simulink model "Muscel_Model"  (R2016b)
settings: Solver=ode45  StartTime=0.0  StopTime=30  FixedStep=0.001  MinStep=0.0001  RelTol=1e-3
libraries: simulink x3
settings Model: Creator=Jan  LastModifiedBy=Jan

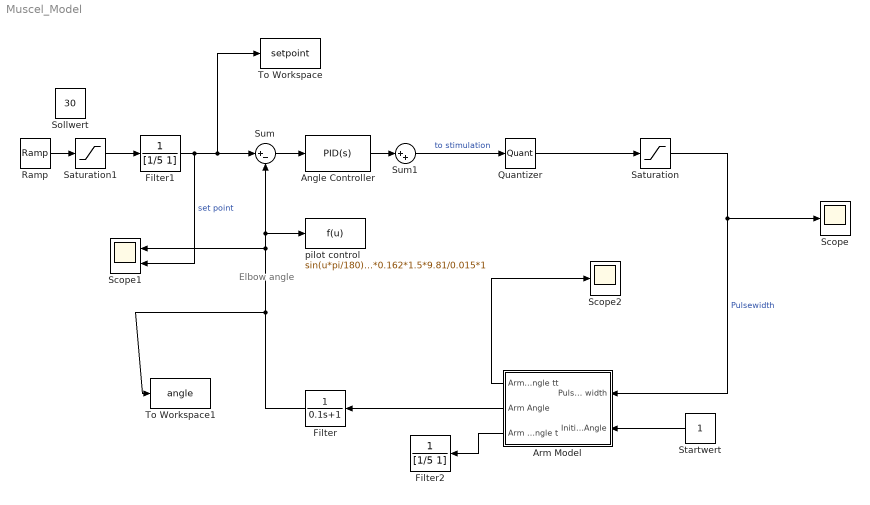
== system Muscel_Model ==
  note: Elbow angle
  Angle Controller : simulink/Continuous/PID Controller  Controller=PID  TimeDomain=Continuous-time  SampleTime=-1  IntegratorMethod=Forward Euler  FilterMethod=Forward Euler  Form=Parallel  UseFilter=on  ControllerParametersSource=internal  P=2  I=2  D=0.1  N=100  InitialConditionSource=internal  InitialConditionForIntegrator=0  InitialConditionForFilter=0  ExternalReset=none  LimitOutput=off  UpperSaturationLimit=500  LowerSaturationLimit=-inf  LinearizeAsGain=on  AntiWindupMode=none  Kb=1  TrackingMode=off  Kt=1  PParamMin=[]  PParamMax=[]  IParamMin=[]  IParamMax=[]  DParamMin=[]  DParamMax=[]  NParamMin=[]  NParamMax=[]  KbParamMin=[]  KbParamMax=[]  KtParamMin=[]  KtParamMax=[]  POutMin=[]  POutMax=[]  IOutMin=[]  IOutMax=[]  DOutMin=[]  DOutMax=[]  NOutMin=[]  NOutMax=[]  KbOutMin=[]  KbOutMax=[]  KtOutMin=[]  KtOutMax=[]  IntegratorOutMin=[]  IntegratorOutMax=[]  FilterOutMin=[]  FilterOutMax=[]  SumOutMin=[]  SumOutMax=[]  SumI1OutMin=[]  SumI1OutMax=[]  SumI2OutMin=[]  SumI2OutMax=[]  SumI3OutMin=[]  SumI3OutMax=[]  SumDOutMin=[]  SumDOutMax=[]  SaturationOutMin=[]  SaturationOutMax=[]  IntegratorContinuousStateAttributes=''  IntegratorStateMustResolveToSignalObject=off  IntegratorRTWStateStorageClass=Auto  FilterContinuousStateAttributes=''  FilterStateMustResolveToSignalObject=off  FilterRTWStateStorageClass=Auto  DifferentiatorICPrevScaledInput=0  DifferentiatorOutMin=[]  DifferentiatorOutMax=[]
  Arm Model : Subsystem
  Filter : TransferFcn  Denominator=[0.1 1]
  Filter1 : TransferFcn  Denominator=[1/5 1]
  Filter2 : TransferFcn  Denominator=[1/5 1]
  Quantizer : Quantizer  QuantizationInterval=10
  Ramp : simulink/Sources/Ramp  slope=5  start=1  X0=0
  Saturation : Saturate  UpperLimit=500  LowerLimit=0
  Saturation1 : Saturate  UpperLimit=40  LowerLimit=0
  Scope : Scope
  Scope1 : Scope  NumInputPorts=2
  Scope2 : Scope
  "Sollwert " : Constant  Value=30
  Startwert : Constant
  Sum : Sum  Inputs=|+-
  Sum1 : Sum  Inputs=|++
  To Workspace : ToWorkspace  VariableName=setpoint  SampleTime=-1
      settings: Save2DSignal=2-D array (concatenate along first dimension)
  To Workspace1 : ToWorkspace  VariableName=angle  SampleTime=-1
      settings: Save2DSignal=2-D array (concatenate along first dimension)
  pilot control : Fcn  Expr=sin(u*pi/180)*0.162*1.5*9.81/0.015*1
  wires:
  Sum/1 -> Angle Controller/1
  Quantizer/1 -> Saturation/1
  Startwert/1 -> Arm Model/2(Initial Angle)
  Saturation/1 -> Arm Model/1(Pulse width), Scope/1  "Pulsewidth"
  Angle Controller/1 -> Sum1/1
  Sum1/1 -> Quantizer/1  "to stimulation"
  Arm Model/2(Arm Angle) -> Filter/1
  Filter/1 -> To Workspace1/1, Scope1/1, pilot control/1, Sum/2
  Filter1/1 -> Scope1/2, To Workspace/1, Sum/1  "set point"
  Arm Model/3(Arm Angle t) -> Filter2/1
  Arm Model/1(Arm Angle tt) -> Scope2/1
  Ramp/1 -> Saturation1/1
  Saturation1/1 -> Filter1/1

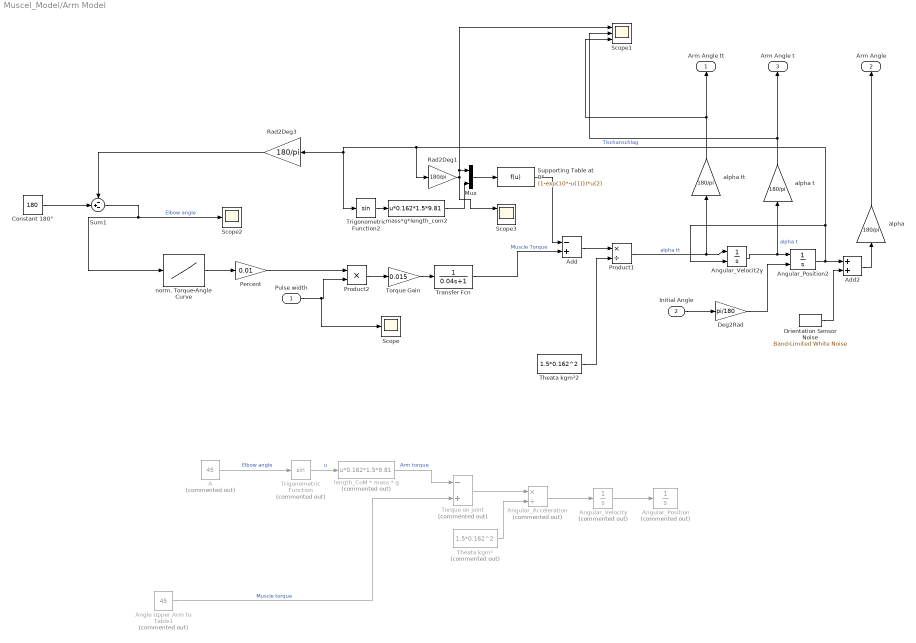
== system Muscel_Model/Arm Model ==
  Pulse width : Inport
  Initial Angle : Inport  Port=2
  A : Constant  Commented=on  Value=45
  Add : Sum  Inputs=-+
  Add2 : Sum
  Angle Upper Arm to Table1 : Constant  Commented=on  Value=45
  Angular_Acceleration : Product  Commented=on  Inputs=*/
  Angular_Position : Integrator  Commented=on  InitialCondition=0.5  LowerSaturationLimit=0
  Angular_Position2 : Integrator  InitialConditionSource=external  InitialCondition=45  LimitOutput=on  UpperSaturationLimit=90*pi/180  LowerSaturationLimit=0
  Angular_Velocit2y : Integrator  ExternalReset=falling
  Angular_Velocity : Integrator  Commented=on
  Constant 180° : Constant  Value=180
  Deg2Rad : Gain  Gain=pi/180
  Mux : Mux  Inputs=2
  Orientation Sensor Noise : simulink/Sources/Band-Limited White Noise  Cov=[0.000001]  Ts=0.01  seed=[23341]
  Percent : Gain  Gain=0.01
  Product1 : Product  Inputs=*/
  Product2 : Product  Inputs=**
  Rad2Deg1 : Gain  Gain=180/pi
  Rad2Deg3 : Gain  Gain=180/pi
  Scope : Scope
  Scope1 : Scope  NumInputPorts=3
  Scope2 : Scope
  Scope3 : Scope  NumInputPorts=3
  Sum1 : Sum  Inputs=-+-
  Supporting Table at 0° : Fcn  Expr=(1-exp(10*-u(1)))*u(2)
  Theata kgm² : Constant  Commented=on  Value=1.5*0.162^2
  Theata kgm²2 : Constant  Value=1.5*0.162^2
  Torque Gain : Gain  Gain=0.015
  Torque on joint : Sum  Commented=on  Inputs=-+
  Transfer Fcn : TransferFcn  Denominator=[0.04 1]
  Trigonometric Function : Trigonometry  Commented=on
  Trigonometric Function2 : Trigonometry
  alpha : Gain  Gain=180/pi
  alpha t : Gain  Gain=180/pi
  alpha tt : Gain  Gain=180/pi
  length_CoM * mass * g : Fcn  Commented=on  Expr=u*0.162*1.5*9.81
  mass*g*length_com2 : Fcn  Expr=u*0.162*1.5*9.81
  norm. Torque-Angle Curve : Lookup_n-D  NumberOfTableDimensions=1  BreakpointsForDimension1=|  Table=|  InternalRulePriority=Speed  RndMeth=Simplest  InputSameDT=on
      BreakpointsForDimension1=|
      | [60.1
      | ;70.1;
      | 80.2;
      | 90.2;
      | 100.2;
      | 110.2
      | ;120.3;
      | 130.3;140.3
      | ;150.4;
      | 160.4]
      Table=|
      | [18;31;47;60;
      | 73;
      | 83
      | ;87;
      | 79;
      | 80;
      | 81
      | ;73]
  Arm Angle tt : Outport
  Arm Angle : Outport  Port=2
  Arm Angle t : Outport  Port=3
  wires:
  Trigonometric Function2/1 -> mass*g*length_com2/1
  norm. Torque-Angle Curve/1 -> Percent/1
  Constant 180°/1 -> Sum1/2
  Sum1/1 -> Scope2/1, norm. Torque-Angle Curve/1  "Elbow angle"
  Theata kgm²2/1 -> Product1/2
  Angular_Velocit2y/1 -> alpha t/1, Angular_Position2/1  "alpha t"
  Add/1 -> Product1/1
  Pulse width/1 -> Scope/1, Product2/2
  Percent/1 -> Product2/1
  Torque Gain/1 -> Transfer Fcn/1
  Product1/1 -> alpha tt/1, Angular_Velocit2y/1  "alpha tt"
  Angular_Position2/1 -> Add2/1, Angular_Velocit2y/2, Rad2Deg1/1, Rad2Deg3/1, Trigonometric Function2/1  "Tischanschlag"
  Deg2Rad/1 -> Angular_Position2/2
  alpha tt/1 -> Scope1/3, Arm Angle tt/1
  Add2/1 -> alpha/1
  alpha/1 -> Arm Angle/1
  Rad2Deg3/1 -> Sum1/1
  Initial Angle/1 -> Deg2Rad/1
  Mux/1 -> Supporting Table at 0°/1
  Rad2Deg1/1 -> Scope3/1, Scope1/1, Mux/1
  Transfer Fcn/1 -> Add/2  "Muscle Torque"
  alpha t/1 -> Arm Angle t/1, Scope1/2
  Orientation Sensor Noise/1 -> Add2/2
  mass*g*length_com2/1 -> Mux/2
  Supporting Table at 0°/1 -> Add/1
  Product2/1 -> Torque Gain/1
  Trigonometric Function/1 -> length_CoM * mass * g/1  "u"
  Theata kgm²/1 -> Angular_Acceleration/2
  Angular_Acceleration/1 -> Angular_Velocity/1
  Angular_Velocity/1 -> Angular_Position/1
  A/1 -> Trigonometric Function/1  "Elbow angle"
  length_CoM * mass * g/1 -> Torque on joint/1  "Arm torque"
  Angle Upper Arm to Table1/1 -> Torque on joint/2  "Muscle torque"
  Torque on joint/1 -> Angular_Acceleration/1
